simulink model "sterowanie1_schemat"  (R2013a)
settings: Solver=ode45  StartTime=0.0  StopTime=10.0  RelTol=1e-3
settings Model: Creator=lukas  LastModifiedBy=lukas

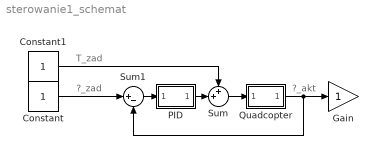
== system sterowanie1_schemat ==
  note: ?_akt
  note: ?_zad
  note: T_zad
  Constant : Constant
  Constant1 : Constant
  Gain : Gain
  PID : Subsystem
  Quadcopter : Subsystem
  Sum : Sum  Inputs=++|
  Sum1 : Sum  Inputs=|+-
  wires:
  Quadcopter/1(Out1) -> Gain/1, Sum1/2
  Sum1/1 -> PID/1(In1)
  Constant/1 -> Sum1/1
  Constant1/1 -> Sum/1
  PID/1(Out1) -> Sum/2
  Sum/1 -> Quadcopter/1(In1)

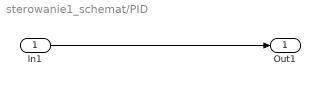
== system sterowanie1_schemat/PID ==
  In1 : Inport
  Out1 : Outport
  wires:
  In1/1 -> Out1/1

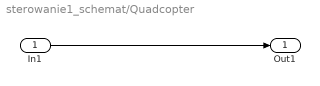
== system sterowanie1_schemat/Quadcopter ==
  In1 : Inport
  Out1 : Outport
  wires:
  In1/1 -> Out1/1
